simulink model "Control_Logic_e"  (R2021a)
settings: Solver=FixedStepAuto  StartTime=Start_time  StopTime=Stop_time  FixedStep=Sample_time  RelTol=1e-3
undefined symbols (not defined in the file or in its folder): Aset_N1, Aset_N10, Aset_N11, Aset_N12, Aset_N2, Aset_N3, Aset_N4, Aset_N5, Aset_N6, Aset_N7, Aset_N8, Aset_N9, Dset_N1, Dset_N2, Sample_time
(part 2 of 3)

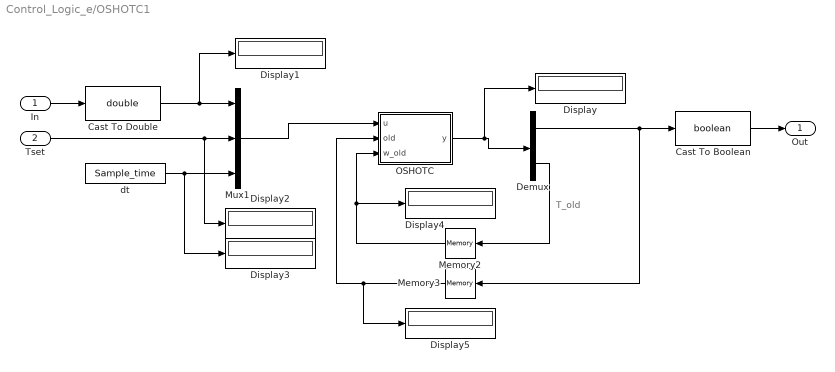
== system Control_Logic_e/OSHOTC1 ==
  note: T_old
  In : Inport
  Tset : Inport  Port=2
  Cast To Boolean : DataTypeConversion  OutDataTypeStr=boolean
  Cast To Double : DataTypeConversion  OutDataTypeStr=double
  Demux : Demux  Outputs=2
  Display{,1..5} (6 alike) : Display
  Memory2 : Memory  InheritSampleTime=on
  Memory3 : Memory  InheritSampleTime=on  LinearizeAsDelay=on
  Mux1 : Mux  Inputs=3
  OSHOTC : MATLAB Function  TreatAsAtomicUnit=on
  dt : Constant  Value=Sample_time  OutDataTypeStr=double  SampleTime=Sample_time
  Out : Outport  VectorParamsAs1DForOutWhenUnconnected=off
  wires:
  OSHOTC/1(y) -> Display/1, Demux/1
  Demux/1 -> Memory3/1, Cast To Boolean/1
  Cast To Boolean/1 -> Out/1
  Mux1/1 -> OSHOTC/1(u)
  Demux/2 -> Memory2/1
  Memory2/1 -> Display4/1, OSHOTC/3(w_old)
  dt/1 -> Display3/1, Mux1/3
  Tset/1 -> Display2/1, Mux1/2
  Memory3/1 -> Display5/1, OSHOTC/2(old)
  In/1 -> Cast To Double/1
  Cast To Double/1 -> Display1/1, Mux1/1

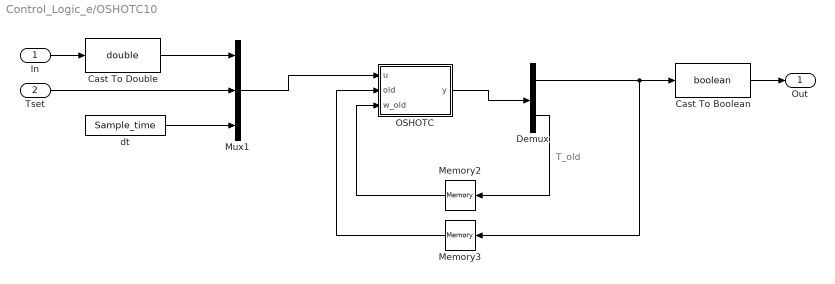
== system Control_Logic_e/OSHOTC10 ==
  note: T_old
  In : Inport
  Tset : Inport  Port=2
  Cast To Boolean : DataTypeConversion  OutDataTypeStr=boolean
  Cast To Double : DataTypeConversion  OutDataTypeStr=double
  Demux : Demux  Outputs=2
  Memory2 : Memory  InheritSampleTime=on
  Memory3 : Memory  InheritSampleTime=on  LinearizeAsDelay=on
  Mux1 : Mux  Inputs=3
  OSHOTC : MATLAB Function  TreatAsAtomicUnit=on
  dt : Constant  Value=Sample_time  OutDataTypeStr=double  SampleTime=Sample_time
  Out : Outport  VectorParamsAs1DForOutWhenUnconnected=off
  wires:
  Cast To Double/1 -> Mux1/1
  In/1 -> Cast To Double/1
  Memory3/1 -> OSHOTC/2(old)
  Tset/1 -> Mux1/2
  dt/1 -> Mux1/3
  Memory2/1 -> OSHOTC/3(w_old)
  Demux/2 -> Memory2/1
  Mux1/1 -> OSHOTC/1(u)
  Cast To Boolean/1 -> Out/1
  Demux/1 -> Cast To Boolean/1, Memory3/1
  OSHOTC/1(y) -> Demux/1

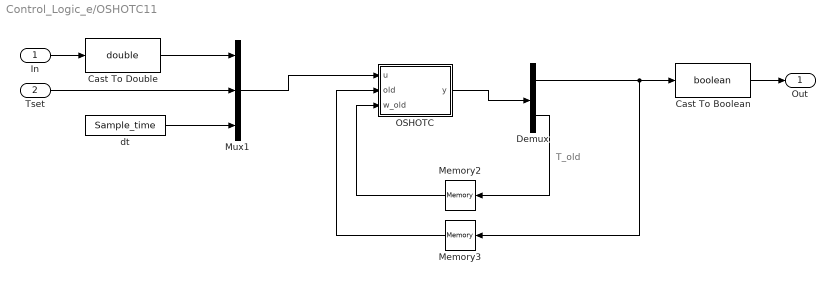
== system Control_Logic_e/OSHOTC11 ==
  note: T_old
  In : Inport
  Tset : Inport  Port=2
  Cast To Boolean : DataTypeConversion  OutDataTypeStr=boolean
  Cast To Double : DataTypeConversion  OutDataTypeStr=double
  Demux : Demux  Outputs=2
  Memory2 : Memory  InheritSampleTime=on
  Memory3 : Memory  InheritSampleTime=on  LinearizeAsDelay=on
  Mux1 : Mux  Inputs=3
  OSHOTC : MATLAB Function  TreatAsAtomicUnit=on
  dt : Constant  Value=Sample_time  OutDataTypeStr=double  SampleTime=Sample_time
  Out : Outport  VectorParamsAs1DForOutWhenUnconnected=off
  wires:
  OSHOTC/1(y) -> Demux/1
  Demux/1 -> Memory3/1, Cast To Boolean/1
  Cast To Boolean/1 -> Out/1
  Mux1/1 -> OSHOTC/1(u)
  Demux/2 -> Memory2/1
  Memory2/1 -> OSHOTC/3(w_old)
  dt/1 -> Mux1/3
  Tset/1 -> Mux1/2
  Memory3/1 -> OSHOTC/2(old)
  In/1 -> Cast To Double/1
  Cast To Double/1 -> Mux1/1

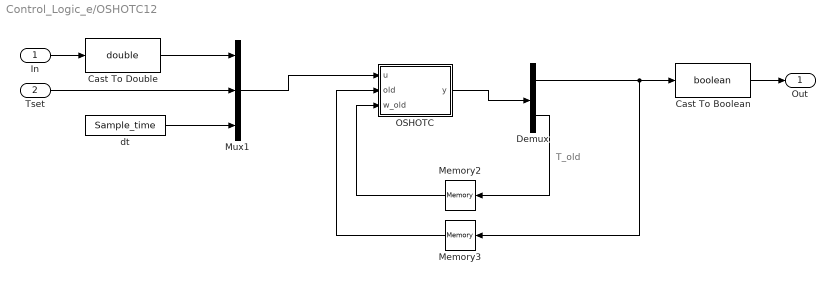
== system Control_Logic_e/OSHOTC12 ==
  note: T_old
  In : Inport
  Tset : Inport  Port=2
  Cast To Boolean : DataTypeConversion  OutDataTypeStr=boolean
  Cast To Double : DataTypeConversion  OutDataTypeStr=double
  Demux : Demux  Outputs=2
  Memory2 : Memory  InheritSampleTime=on
  Memory3 : Memory  InheritSampleTime=on  LinearizeAsDelay=on
  Mux1 : Mux  Inputs=3
  OSHOTC : MATLAB Function  TreatAsAtomicUnit=on
  dt : Constant  Value=Sample_time  OutDataTypeStr=double  SampleTime=Sample_time
  Out : Outport  VectorParamsAs1DForOutWhenUnconnected=off
  wires:
  OSHOTC/1(y) -> Demux/1
  Demux/1 -> Memory3/1, Cast To Boolean/1
  Cast To Boolean/1 -> Out/1
  Mux1/1 -> OSHOTC/1(u)
  Demux/2 -> Memory2/1
  Memory2/1 -> OSHOTC/3(w_old)
  dt/1 -> Mux1/3
  Tset/1 -> Mux1/2
  Memory3/1 -> OSHOTC/2(old)
  In/1 -> Cast To Double/1
  Cast To Double/1 -> Mux1/1

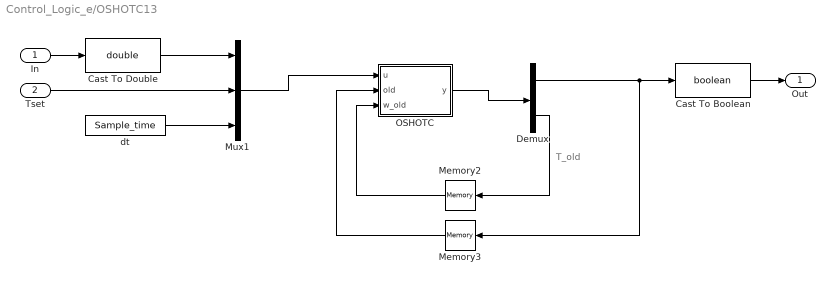
== system Control_Logic_e/OSHOTC13 ==
  note: T_old
  In : Inport
  Tset : Inport  Port=2
  Cast To Boolean : DataTypeConversion  OutDataTypeStr=boolean
  Cast To Double : DataTypeConversion  OutDataTypeStr=double
  Demux : Demux  Outputs=2
  Memory2 : Memory  InheritSampleTime=on
  Memory3 : Memory  InheritSampleTime=on  LinearizeAsDelay=on
  Mux1 : Mux  Inputs=3
  OSHOTC : MATLAB Function  TreatAsAtomicUnit=on
  dt : Constant  Value=Sample_time  OutDataTypeStr=double  SampleTime=Sample_time
  Out : Outport  VectorParamsAs1DForOutWhenUnconnected=off
  wires:
  OSHOTC/1(y) -> Demux/1
  Demux/1 -> Memory3/1, Cast To Boolean/1
  Cast To Boolean/1 -> Out/1
  Mux1/1 -> OSHOTC/1(u)
  Demux/2 -> Memory2/1
  Memory2/1 -> OSHOTC/3(w_old)
  dt/1 -> Mux1/3
  Tset/1 -> Mux1/2
  Memory3/1 -> OSHOTC/2(old)
  In/1 -> Cast To Double/1
  Cast To Double/1 -> Mux1/1

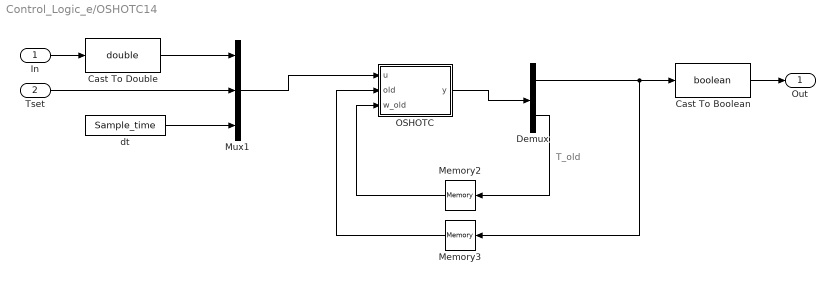
== system Control_Logic_e/OSHOTC14 ==
  note: T_old
  In : Inport
  Tset : Inport  Port=2
  Cast To Boolean : DataTypeConversion  OutDataTypeStr=boolean
  Cast To Double : DataTypeConversion  OutDataTypeStr=double
  Demux : Demux  Outputs=2
  Memory2 : Memory  InheritSampleTime=on
  Memory3 : Memory  InheritSampleTime=on  LinearizeAsDelay=on
  Mux1 : Mux  Inputs=3
  OSHOTC : MATLAB Function  TreatAsAtomicUnit=on
  dt : Constant  Value=Sample_time  OutDataTypeStr=double  SampleTime=Sample_time
  Out : Outport  VectorParamsAs1DForOutWhenUnconnected=off
  wires:
  OSHOTC/1(y) -> Demux/1
  Demux/1 -> Memory3/1, Cast To Boolean/1
  Cast To Boolean/1 -> Out/1
  Mux1/1 -> OSHOTC/1(u)
  Demux/2 -> Memory2/1
  Memory2/1 -> OSHOTC/3(w_old)
  dt/1 -> Mux1/3
  Tset/1 -> Mux1/2
  Memory3/1 -> OSHOTC/2(old)
  In/1 -> Cast To Double/1
  Cast To Double/1 -> Mux1/1

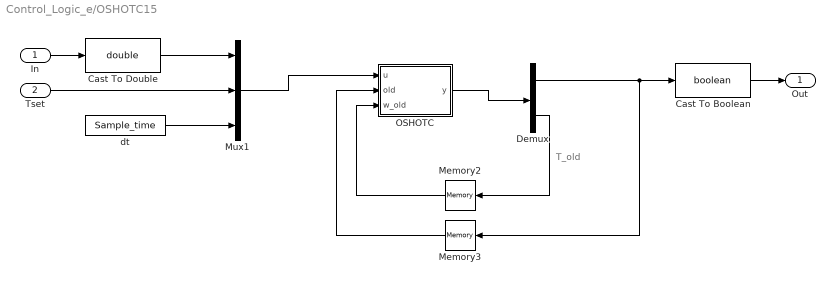
== system Control_Logic_e/OSHOTC15 ==
  note: T_old
  In : Inport
  Tset : Inport  Port=2
  Cast To Boolean : DataTypeConversion  OutDataTypeStr=boolean
  Cast To Double : DataTypeConversion  OutDataTypeStr=double
  Demux : Demux  Outputs=2
  Memory2 : Memory  InheritSampleTime=on
  Memory3 : Memory  InheritSampleTime=on  LinearizeAsDelay=on
  Mux1 : Mux  Inputs=3
  OSHOTC : MATLAB Function  TreatAsAtomicUnit=on
  dt : Constant  Value=Sample_time  OutDataTypeStr=double  SampleTime=Sample_time
  Out : Outport  VectorParamsAs1DForOutWhenUnconnected=off
  wires:
  OSHOTC/1(y) -> Demux/1
  Demux/1 -> Memory3/1, Cast To Boolean/1
  Cast To Boolean/1 -> Out/1
  Mux1/1 -> OSHOTC/1(u)
  Demux/2 -> Memory2/1
  Memory2/1 -> OSHOTC/3(w_old)
  dt/1 -> Mux1/3
  Tset/1 -> Mux1/2
  Memory3/1 -> OSHOTC/2(old)
  In/1 -> Cast To Double/1
  Cast To Double/1 -> Mux1/1

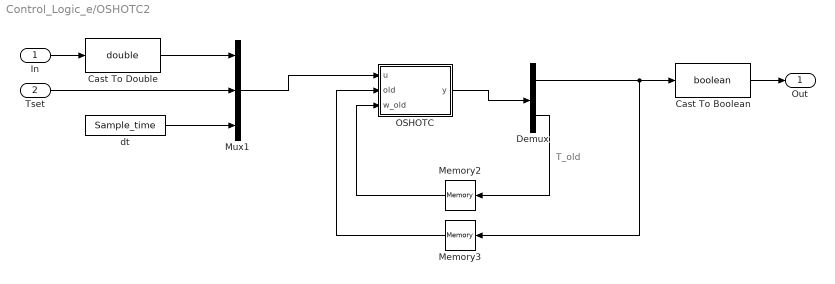
== system Control_Logic_e/OSHOTC2 ==
  note: T_old
  In : Inport
  Tset : Inport  Port=2
  Cast To Boolean : DataTypeConversion  OutDataTypeStr=boolean
  Cast To Double : DataTypeConversion  OutDataTypeStr=double
  Demux : Demux  Outputs=2
  Memory2 : Memory  InheritSampleTime=on
  Memory3 : Memory  InheritSampleTime=on  LinearizeAsDelay=on
  Mux1 : Mux  Inputs=3
  OSHOTC : MATLAB Function  TreatAsAtomicUnit=on
  dt : Constant  Value=Sample_time  OutDataTypeStr=double  SampleTime=Sample_time
  Out : Outport  VectorParamsAs1DForOutWhenUnconnected=off
  wires:
  OSHOTC/1(y) -> Demux/1
  Demux/1 -> Memory3/1, Cast To Boolean/1
  Cast To Boolean/1 -> Out/1
  Mux1/1 -> OSHOTC/1(u)
  Demux/2 -> Memory2/1
  Memory2/1 -> OSHOTC/3(w_old)
  dt/1 -> Mux1/3
  Tset/1 -> Mux1/2
  Memory3/1 -> OSHOTC/2(old)
  In/1 -> Cast To Double/1
  Cast To Double/1 -> Mux1/1

== system Control_Logic_e/OSHOTC3 ==
  note: T_old
  In : Inport
  Tset : Inport  Port=2
  Cast To Boolean : DataTypeConversion  OutDataTypeStr=boolean
  Cast To Double : DataTypeConversion  OutDataTypeStr=double
  Demux : Demux  Outputs=2
  Memory2 : Memory  InheritSampleTime=on
  Memory3 : Memory  InheritSampleTime=on  LinearizeAsDelay=on
  Mux1 : Mux  Inputs=3
  OSHOTC : MATLAB Function  TreatAsAtomicUnit=on
  dt : Constant  Value=Sample_time  OutDataTypeStr=double  SampleTime=Sample_time
  Out : Outport  VectorParamsAs1DForOutWhenUnconnected=off
  wires:
  OSHOTC/1(y) -> Demux/1
  Demux/1 -> Memory3/1, Cast To Boolean/1
  Cast To Boolean/1 -> Out/1
  Mux1/1 -> OSHOTC/1(u)
  Demux/2 -> Memory2/1
  Memory2/1 -> OSHOTC/3(w_old)
  dt/1 -> Mux1/3
  Tset/1 -> Mux1/2
  Memory3/1 -> OSHOTC/2(old)
  In/1 -> Cast To Double/1
  Cast To Double/1 -> Mux1/1

== system Control_Logic_e/OSHOTC4 ==
  note: T_old
  In : Inport
  Tset : Inport  Port=2
  Cast To Boolean : DataTypeConversion  OutDataTypeStr=boolean
  Cast To Double : DataTypeConversion  OutDataTypeStr=double
  Demux : Demux  Outputs=2
  Memory2 : Memory  InheritSampleTime=on
  Memory3 : Memory  InheritSampleTime=on  LinearizeAsDelay=on
  Mux1 : Mux  Inputs=3
  OSHOTC : MATLAB Function  TreatAsAtomicUnit=on
  dt : Constant  Value=Sample_time  OutDataTypeStr=double  SampleTime=Sample_time
  Out : Outport  VectorParamsAs1DForOutWhenUnconnected=off
  wires:
  OSHOTC/1(y) -> Demux/1
  Demux/1 -> Memory3/1, Cast To Boolean/1
  Cast To Boolean/1 -> Out/1
  Mux1/1 -> OSHOTC/1(u)
  Demux/2 -> Memory2/1
  Memory2/1 -> OSHOTC/3(w_old)
  dt/1 -> Mux1/3
  Tset/1 -> Mux1/2
  Memory3/1 -> OSHOTC/2(old)
  In/1 -> Cast To Double/1
  Cast To Double/1 -> Mux1/1

== system Control_Logic_e/OSHOTC5 ==
  note: T_old
  In : Inport
  Tset : Inport  Port=2
  Cast To Boolean : DataTypeConversion  OutDataTypeStr=boolean
  Cast To Double : DataTypeConversion  OutDataTypeStr=double
  Demux : Demux  Outputs=2
  Memory2 : Memory  InheritSampleTime=on
  Memory3 : Memory  InheritSampleTime=on  LinearizeAsDelay=on
  Mux1 : Mux  Inputs=3
  OSHOTC : MATLAB Function  TreatAsAtomicUnit=on
  dt : Constant  Value=Sample_time  OutDataTypeStr=double  SampleTime=Sample_time
  Out : Outport  VectorParamsAs1DForOutWhenUnconnected=off
  wires:
  OSHOTC/1(y) -> Demux/1
  Demux/1 -> Memory3/1, Cast To Boolean/1
  Cast To Boolean/1 -> Out/1
  Mux1/1 -> OSHOTC/1(u)
  Demux/2 -> Memory2/1
  Memory2/1 -> OSHOTC/3(w_old)
  dt/1 -> Mux1/3
  Tset/1 -> Mux1/2
  Memory3/1 -> OSHOTC/2(old)
  In/1 -> Cast To Double/1
  Cast To Double/1 -> Mux1/1

== system Control_Logic_e/OSHOTC6 ==
  note: T_old
  In : Inport
  Tset : Inport  Port=2
  Cast To Boolean : DataTypeConversion  OutDataTypeStr=boolean
  Cast To Double : DataTypeConversion  OutDataTypeStr=double
  Demux : Demux  Outputs=2
  Memory2 : Memory  InheritSampleTime=on
  Memory3 : Memory  InheritSampleTime=on  LinearizeAsDelay=on
  Mux1 : Mux  Inputs=3
  OSHOTC : MATLAB Function  TreatAsAtomicUnit=on
  dt : Constant  Value=Sample_time  OutDataTypeStr=double  SampleTime=Sample_time
  Out : Outport  VectorParamsAs1DForOutWhenUnconnected=off
  wires:
  OSHOTC/1(y) -> Demux/1
  Demux/1 -> Memory3/1, Cast To Boolean/1
  Cast To Boolean/1 -> Out/1
  Mux1/1 -> OSHOTC/1(u)
  Demux/2 -> Memory2/1
  Memory2/1 -> OSHOTC/3(w_old)
  dt/1 -> Mux1/3
  Tset/1 -> Mux1/2
  Memory3/1 -> OSHOTC/2(old)
  In/1 -> Cast To Double/1
  Cast To Double/1 -> Mux1/1

== system Control_Logic_e/OSHOTC7 ==
  note: T_old
  In : Inport
  Tset : Inport  Port=2
  Cast To Boolean : DataTypeConversion  OutDataTypeStr=boolean
  Cast To Double : DataTypeConversion  OutDataTypeStr=double
  Demux : Demux  Outputs=2
  Memory2 : Memory  InheritSampleTime=on
  Memory3 : Memory  InheritSampleTime=on  LinearizeAsDelay=on
  Mux1 : Mux  Inputs=3
  OSHOTC : MATLAB Function  TreatAsAtomicUnit=on
  dt : Constant  Value=Sample_time  OutDataTypeStr=double  SampleTime=Sample_time
  Out : Outport  VectorParamsAs1DForOutWhenUnconnected=off
  wires:
  OSHOTC/1(y) -> Demux/1
  Demux/1 -> Memory3/1, Cast To Boolean/1
  Cast To Boolean/1 -> Out/1
  Mux1/1 -> OSHOTC/1(u)
  Demux/2 -> Memory2/1
  Memory2/1 -> OSHOTC/3(w_old)
  dt/1 -> Mux1/3
  Tset/1 -> Mux1/2
  Memory3/1 -> OSHOTC/2(old)
  In/1 -> Cast To Double/1
  Cast To Double/1 -> Mux1/1

== system Control_Logic_e/OSHOTC8 ==
  note: T_old
  In : Inport
  Tset : Inport  Port=2
  Cast To Boolean : DataTypeConversion  OutDataTypeStr=boolean
  Cast To Double : DataTypeConversion  OutDataTypeStr=double
  Demux : Demux  Outputs=2
  Memory2 : Memory  InheritSampleTime=on
  Memory3 : Memory  InheritSampleTime=on  LinearizeAsDelay=on
  Mux1 : Mux  Inputs=3
  OSHOTC : MATLAB Function  TreatAsAtomicUnit=on
  dt : Constant  Value=Sample_time  OutDataTypeStr=double  SampleTime=Sample_time
  Out : Outport  VectorParamsAs1DForOutWhenUnconnected=off
  wires:
  OSHOTC/1(y) -> Demux/1
  Demux/1 -> Memory3/1, Cast To Boolean/1
  Cast To Boolean/1 -> Out/1
  Mux1/1 -> OSHOTC/1(u)
  Demux/2 -> Memory2/1
  Memory2/1 -> OSHOTC/3(w_old)
  dt/1 -> Mux1/3
  Tset/1 -> Mux1/2
  Memory3/1 -> OSHOTC/2(old)
  In/1 -> Cast To Double/1
  Cast To Double/1 -> Mux1/1

== system Control_Logic_e/OSHOTC9 ==
  note: T_old
  In : Inport
  Tset : Inport  Port=2
  Cast To Boolean : DataTypeConversion  OutDataTypeStr=boolean
  Cast To Double : DataTypeConversion  OutDataTypeStr=double
  Demux : Demux  Outputs=2
  Memory2 : Memory  InheritSampleTime=on
  Memory3 : Memory  InheritSampleTime=on  LinearizeAsDelay=on
  Mux1 : Mux  Inputs=3
  OSHOTC : MATLAB Function  TreatAsAtomicUnit=on
  dt : Constant  Value=Sample_time  OutDataTypeStr=double  SampleTime=Sample_time
  Out : Outport  VectorParamsAs1DForOutWhenUnconnected=off
  wires:
  OSHOTC/1(y) -> Demux/1
  Demux/1 -> Memory3/1, Cast To Boolean/1
  Cast To Boolean/1 -> Out/1
  Mux1/1 -> OSHOTC/1(u)
  Demux/2 -> Memory2/1
  Memory2/1 -> OSHOTC/3(w_old)
  dt/1 -> Mux1/3
  Tset/1 -> Mux1/2
  Memory3/1 -> OSHOTC/2(old)
  In/1 -> Cast To Double/1
  Cast To Double/1 -> Mux1/1

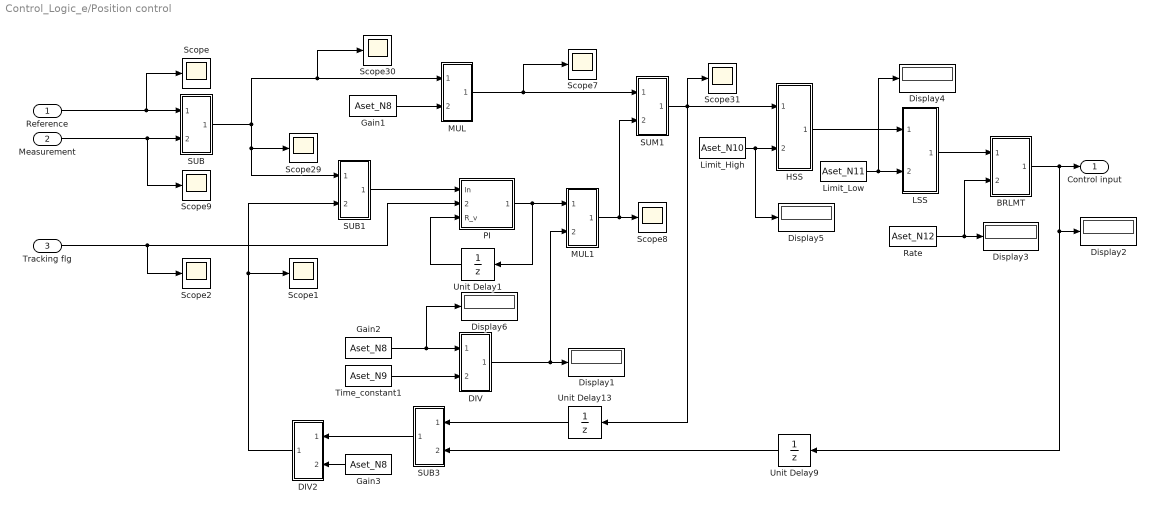
== system Control_Logic_e/Position control ==
  Reference : Inport
  Measurement : Inport  Port=2
  Tracking flg : Inport  Port=3
  BRLMT : Subsystem
  DIV : Subsystem
  DIV2 : Subsystem
  Display{1..6} (6 alike) : Display
  Gain1 : Constant  Value=Aset_N8  OutDataTypeStr=double  SampleTime=Sample_time
  Gain2 : Constant  Value=Aset_N8  OutDataTypeStr=double  SampleTime=Sample_time
  Gain3 : Constant  Value=Aset_N8  OutDataTypeStr=double  SampleTime=Sample_time
  HSS : Subsystem
  LSS : Subsystem
  Limit_High : Constant  Value=Aset_N10  OutDataTypeStr=double  SampleTime=Sample_time
  Limit_Low : Constant  Value=Aset_N11  OutDataTypeStr=double  SampleTime=Sample_time
  MUL : Subsystem
  MUL1 : Subsystem
  PI : Subsystem
  Rate : Constant  Value=Aset_N12  OutDataTypeStr=double  SampleTime=Sample_time
  SUB : Subsystem
  SUB1 : Subsystem
  SUB3 : Subsystem
  SUM1 : Subsystem
  Scope{,1..2,7..9,29..31} (9 alike) : Scope
  Time_constant1 : Constant  Value=Aset_N9  OutDataTypeStr=double  SampleTime=Sample_time
  Unit Delay1 : UnitDelay  SampleTime=Sample_time  HasFrameUpgradeWarning=on
  Unit Delay13 : UnitDelay  SampleTime=Sample_time  HasFrameUpgradeWarning=on
  Unit Delay9 : UnitDelay  SampleTime=Sample_time  HasFrameUpgradeWarning=on
  Control input : Outport  VectorParamsAs1DForOutWhenUnconnected=off
  wires:
  SUM1/1(Out) -> HSS/1(In1), Unit Delay13/1, Scope31/1
  Measurement/1 -> SUB/2(In2), Scope9/1
  SUB/1(Out) -> Scope30/1, MUL/1(In1), SUB1/1(In1), Scope29/1
  Unit Delay13/1 -> SUB3/1(In1)
  MUL/1(Out) -> Scope7/1, SUM1/1(In1)
  SUB3/1(Out) -> DIV2/1(In1)
  SUB1/1(Out) -> PI/1(In)
  Gain1/1 -> MUL/2(In2)
  LSS/1(Out1) -> BRLMT/1(In1)
  Reference/1 -> SUB/1(In1), Scope/1
  Gain3/1 -> DIV2/2(In2)
  Limit_Low/1 -> LSS/2(In2), Display4/1
  Tracking flg/1 -> PI/2(Reset), Scope2/1
  PI/1(Out1) -> MUL1/1(In1), Unit Delay1/1
  Limit_High/1 -> HSS/2(In2), Display5/1
  MUL1/1(Out) -> SUM1/2(In2), Scope8/1
  BRLMT/1(Out1) -> Unit Delay9/1, Display2/1, Control input/1
  Time_constant1/1 -> DIV/2(In2)
  Gain2/1 -> DIV/1(In1), Display6/1
  HSS/1(Out1) -> LSS/1(In1)
  DIV2/1(Out1) -> SUB1/2(In2), Scope1/1
  Unit Delay9/1 -> SUB3/2(In2)
  DIV/1(Out1) -> MUL1/2(In2), Display1/1
  Rate/1 -> BRLMT/2(In2), Display3/1
  Unit Delay1/1 -> PI/3(R_v)

== system Control_Logic_e/SUB ==
  In1 : Inport
  In2 : Inport  Port=2
  Mux : Mux  Inputs=2
  SUB : MATLAB Function  TreatAsAtomicUnit=on
  Out : Outport  VectorParamsAs1DForOutWhenUnconnected=off
  wires:
  In2/1 -> Mux/2
  SUB/1(y) -> Out/1
  Mux/1 -> SUB/1(u)
  In1/1 -> Mux/1

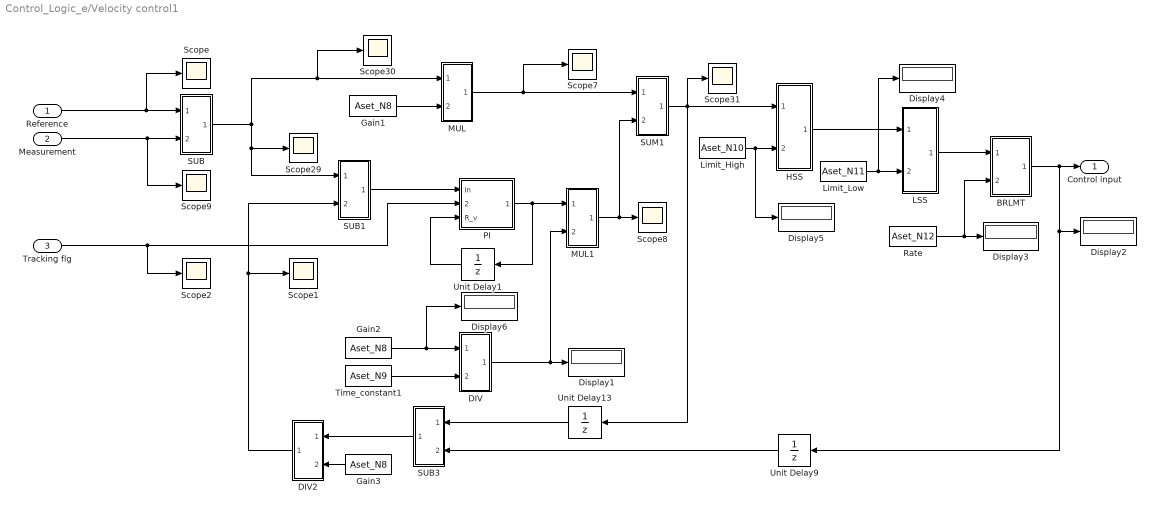
== system Control_Logic_e/Velocity control1 ==
  Reference : Inport
  Measurement : Inport  Port=2
  Tracking flg : Inport  Port=3
  BRLMT : Subsystem
  DIV : Subsystem
  DIV2 : Subsystem
  Display{1..6} (6 alike) : Display
  Gain1 : Constant  Value=Aset_N8  OutDataTypeStr=double  SampleTime=Sample_time
  Gain2 : Constant  Value=Aset_N8  OutDataTypeStr=double  SampleTime=Sample_time
  Gain3 : Constant  Value=Aset_N8  OutDataTypeStr=double  SampleTime=Sample_time
  HSS : Subsystem
  LSS : Subsystem
  Limit_High : Constant  Value=Aset_N10  OutDataTypeStr=double  SampleTime=Sample_time
  Limit_Low : Constant  Value=Aset_N11  OutDataTypeStr=double  SampleTime=Sample_time
  MUL : Subsystem
  MUL1 : Subsystem
  PI : Subsystem
  Rate : Constant  Value=Aset_N12  OutDataTypeStr=double  SampleTime=Sample_time
  SUB : Subsystem
  SUB1 : Subsystem
  SUB3 : Subsystem
  SUM1 : Subsystem
  Scope{,1..2,7..9,29..31} (9 alike) : Scope
  Time_constant1 : Constant  Value=Aset_N9  OutDataTypeStr=double  SampleTime=Sample_time
  Unit Delay1 : UnitDelay  SampleTime=Sample_time  HasFrameUpgradeWarning=on
  Unit Delay13 : UnitDelay  SampleTime=Sample_time  HasFrameUpgradeWarning=on
  Unit Delay9 : UnitDelay  SampleTime=Sample_time  HasFrameUpgradeWarning=on
  Control input : Outport  VectorParamsAs1DForOutWhenUnconnected=off
  wires:
  Unit Delay1/1 -> PI/3(R_v)
  Rate/1 -> Display3/1, BRLMT/2(In2)
  DIV/1(Out1) -> Display1/1, MUL1/2(In2)
  Unit Delay9/1 -> SUB3/2(In2)
  DIV2/1(Out1) -> Scope1/1, SUB1/2(In2)
  HSS/1(Out1) -> LSS/1(In1)
  Gain2/1 -> Display6/1, DIV/1(In1)
  Time_constant1/1 -> DIV/2(In2)
  BRLMT/1(Out1) -> Control input/1, Display2/1, Unit Delay9/1
  MUL1/1(Out) -> Scope8/1, SUM1/2(In2)
  Limit_High/1 -> Display5/1, HSS/2(In2)
  PI/1(Out1) -> Unit Delay1/1, MUL1/1(In1)
  Tracking flg/1 -> Scope2/1, PI/2(Reset)
  Limit_Low/1 -> Display4/1, LSS/2(In2)
  Gain3/1 -> DIV2/2(In2)
  Reference/1 -> Scope/1, SUB/1(In1)
  LSS/1(Out1) -> BRLMT/1(In1)
  Gain1/1 -> MUL/2(In2)
  SUB1/1(Out) -> PI/1(In)
  SUB3/1(Out) -> DIV2/1(In1)
  MUL/1(Out) -> SUM1/1(In1), Scope7/1
  Unit Delay13/1 -> SUB3/1(In1)
  SUB/1(Out) -> Scope29/1, SUB1/1(In1), MUL/1(In1), Scope30/1
  Measurement/1 -> Scope9/1, SUB/2(In2)
  SUM1/1(Out) -> Scope31/1, Unit Delay13/1, HSS/1(In1)

== system Control_Logic_e/Position control/BRLMT ==
  In1 : Inport
  In2 : Inport  Port=2
  BRLMT : MATLAB Function  TreatAsAtomicUnit=on
  Display : Display
  Memory : Memory  InheritSampleTime=on  LinearizeMemory=on  LinearizeAsDelay=on
  Mux1 : Mux  Inputs=3
  dt : Constant  Value=Sample_time  OutDataTypeStr=double  SampleTime=Sample_time
  Out1 : Outport  VectorParamsAs1DForOutWhenUnconnected=off
  wires:
  In1/1 -> Mux1/1
  Mux1/1 -> Display/1, BRLMT/1(u)
  BRLMT/1(y) -> Out1/1, Memory/1
  Memory/1 -> BRLMT/2(old)
  In2/1 -> Mux1/2
  dt/1 -> Mux1/3

== system Control_Logic_e/Position control/DIV ==
  In1 : Inport
  In2 : Inport  Port=2
  DIV : MATLAB Function  TreatAsAtomicUnit=on
  Display : Display
  Display1 : Display
  FlowMax1 : Constant  Value=3.402823e+38  OutDataTypeStr=double  SampleTime=Sample_time
  Mux : Mux  Inputs=3
  Out1 : Outport  VectorParamsAs1DForOutWhenUnconnected=off
  wires:
  FlowMax1/1 -> Mux/3
  In1/1 -> Mux/1, Display/1
  Mux/1 -> DIV/1(u)
  DIV/1(y) -> Out1/1
  In2/1 -> Display1/1, Mux/2

== system Control_Logic_e/Position control/DIV2 ==
  In1 : Inport
  In2 : Inport  Port=2
  DIV : MATLAB Function  TreatAsAtomicUnit=on
  Display : Display
  Display1 : Display
  FlowMax1 : Constant  Value=3.402823e+38  OutDataTypeStr=double  SampleTime=Sample_time
  Mux : Mux  Inputs=3
  Out1 : Outport  VectorParamsAs1DForOutWhenUnconnected=off
  wires:
  FlowMax1/1 -> Mux/3
  In1/1 -> Mux/1, Display/1
  Mux/1 -> DIV/1(u)
  DIV/1(y) -> Out1/1
  In2/1 -> Display1/1, Mux/2

== system Control_Logic_e/Position control/HSS ==
  In1 : Inport
  In2 : Inport  Port=2
  HSS : MATLAB Function  TreatAsAtomicUnit=on
  Mux : Mux  Inputs=2
  Out1 : Outport  VectorParamsAs1DForOutWhenUnconnected=off
  wires:
  HSS/1(y) -> Out1/1
  In1/1 -> Mux/1
  In2/1 -> Mux/2
  Mux/1 -> HSS/1(u)

== system Control_Logic_e/Position control/LSS ==
  In1 : Inport
  In2 : Inport  Port=2
  LSS : MATLAB Function  TreatAsAtomicUnit=on
  Mux : Mux  Inputs=2
  Out1 : Outport  VectorParamsAs1DForOutWhenUnconnected=off
  wires:
  LSS/1(y) -> Out1/1
  Mux/1 -> LSS/1(u)
  In1/1 -> Mux/1
  In2/1 -> Mux/2

== system Control_Logic_e/Position control/MUL ==
  In1 : Inport
  In2 : Inport  Port=2
  MUL : MATLAB Function  TreatAsAtomicUnit=on
  Mux : Mux  Inputs=2
  Out : Outport  VectorParamsAs1DForOutWhenUnconnected=off
  wires:
  In1/1 -> Mux/1
  Mux/1 -> MUL/1(u)
  MUL/1(y) -> Out/1
  In2/1 -> Mux/2

== system Control_Logic_e/Position control/MUL1 ==
  In1 : Inport
  In2 : Inport  Port=2
  MUL : MATLAB Function  TreatAsAtomicUnit=on
  Mux : Mux  Inputs=2
  Out : Outport  VectorParamsAs1DForOutWhenUnconnected=off
  wires:
  In1/1 -> Mux/1
  Mux/1 -> MUL/1(u)
  MUL/1(y) -> Out/1
  In2/1 -> Mux/2

== system Control_Logic_e/Position control/PI ==
  In : Inport
  Reset : Inport  Port=2
  R_v : Inport  Port=3
  Cast To Double : DataTypeConversion  OutDataTypeStr=double
  Memory : Memory  InheritSampleTime=on
  Mux : Mux
  PI : MATLAB Function  TreatAsAtomicUnit=on
  dt : Constant  Value=Sample_time  OutDataTypeStr=double  SampleTime=Sample_time
  Out1 : Outport  VectorParamsAs1DForOutWhenUnconnected=off
  wires:
  In/1 -> Mux/1
  Reset/1 -> Cast To Double/1
  PI/1(y) -> Out1/1, Memory/1
  Mux/1 -> PI/1(u)
  R_v/1 -> Mux/3
  dt/1 -> Mux/4
  Cast To Double/1 -> Mux/2
  Memory/1 -> PI/2(old)

== system Control_Logic_e/Position control/SUB ==
  In1 : Inport
  In2 : Inport  Port=2
  Mux : Mux  Inputs=2
  SUB : MATLAB Function  TreatAsAtomicUnit=on
  Out : Outport  VectorParamsAs1DForOutWhenUnconnected=off
  wires:
  In2/1 -> Mux/2
  SUB/1(y) -> Out/1
  Mux/1 -> SUB/1(u)
  In1/1 -> Mux/1

== system Control_Logic_e/Position control/SUB1 ==
  In1 : Inport
  In2 : Inport  Port=2
  Mux : Mux  Inputs=2
  SUB : MATLAB Function  TreatAsAtomicUnit=on
  Out : Outport  VectorParamsAs1DForOutWhenUnconnected=off
  wires:
  In1/1 -> Mux/1
  Mux/1 -> SUB/1(u)
  SUB/1(y) -> Out/1
  In2/1 -> Mux/2

== system Control_Logic_e/Position control/SUB3 ==
  In1 : Inport
  In2 : Inport  Port=2
  Mux : Mux  Inputs=2
  SUB : MATLAB Function  TreatAsAtomicUnit=on
  Out : Outport  VectorParamsAs1DForOutWhenUnconnected=off
  wires:
  In2/1 -> Mux/2
  SUB/1(y) -> Out/1
  Mux/1 -> SUB/1(u)
  In1/1 -> Mux/1

== system Control_Logic_e/Position control/SUM1 ==
  In1 : Inport
  In2 : Inport  Port=2
  Mux : Mux  Inputs=2
  SUM : MATLAB Function  TreatAsAtomicUnit=on
  Out : Outport  VectorParamsAs1DForOutWhenUnconnected=off
  wires:
  Mux/1 -> SUM/1(u)
  SUM/1(y) -> Out/1
  In1/1 -> Mux/1
  In2/1 -> Mux/2

== system Control_Logic_e/Velocity control1/BRLMT ==
  In1 : Inport
  In2 : Inport  Port=2
  BRLMT : MATLAB Function  TreatAsAtomicUnit=on
  Display : Display
  Memory : Memory  InheritSampleTime=on  LinearizeMemory=on  LinearizeAsDelay=on
  Mux1 : Mux  Inputs=3
  dt : Constant  Value=Sample_time  OutDataTypeStr=double  SampleTime=Sample_time
  Out1 : Outport  VectorParamsAs1DForOutWhenUnconnected=off
  wires:
  dt/1 -> Mux1/3
  In2/1 -> Mux1/2
  Memory/1 -> BRLMT/2(old)
  BRLMT/1(y) -> Memory/1, Out1/1
  Mux1/1 -> BRLMT/1(u), Display/1
  In1/1 -> Mux1/1

== system Control_Logic_e/Velocity control1/DIV ==
  In1 : Inport
  In2 : Inport  Port=2
  DIV : MATLAB Function  TreatAsAtomicUnit=on
  Display : Display
  Display1 : Display
  FlowMax1 : Constant  Value=3.402823e+38  OutDataTypeStr=double  SampleTime=Sample_time
  Mux : Mux  Inputs=3
  Out1 : Outport  VectorParamsAs1DForOutWhenUnconnected=off
  wires:
  In2/1 -> Mux/2, Display1/1
  DIV/1(y) -> Out1/1
  Mux/1 -> DIV/1(u)
  In1/1 -> Display/1, Mux/1
  FlowMax1/1 -> Mux/3

== system Control_Logic_e/Velocity control1/DIV2 ==
  In1 : Inport
  In2 : Inport  Port=2
  DIV : MATLAB Function  TreatAsAtomicUnit=on
  Display : Display
  Display1 : Display
  FlowMax1 : Constant  Value=3.402823e+38  OutDataTypeStr=double  SampleTime=Sample_time
  Mux : Mux  Inputs=3
  Out1 : Outport  VectorParamsAs1DForOutWhenUnconnected=off
  wires:
  In2/1 -> Mux/2, Display1/1
  DIV/1(y) -> Out1/1
  Mux/1 -> DIV/1(u)
  In1/1 -> Display/1, Mux/1
  FlowMax1/1 -> Mux/3

== system Control_Logic_e/Velocity control1/HSS ==
  In1 : Inport
  In2 : Inport  Port=2
  HSS : MATLAB Function  TreatAsAtomicUnit=on
  Mux : Mux  Inputs=2
  Out1 : Outport  VectorParamsAs1DForOutWhenUnconnected=off
  wires:
  Mux/1 -> HSS/1(u)
  In2/1 -> Mux/2
  In1/1 -> Mux/1
  HSS/1(y) -> Out1/1

== system Control_Logic_e/Velocity control1/LSS ==
  In1 : Inport
  In2 : Inport  Port=2
  LSS : MATLAB Function  TreatAsAtomicUnit=on
  Mux : Mux  Inputs=2
  Out1 : Outport  VectorParamsAs1DForOutWhenUnconnected=off
  wires:
  In2/1 -> Mux/2
  In1/1 -> Mux/1
  Mux/1 -> LSS/1(u)
  LSS/1(y) -> Out1/1

== system Control_Logic_e/Velocity control1/MUL ==
  In1 : Inport
  In2 : Inport  Port=2
  MUL : MATLAB Function  TreatAsAtomicUnit=on
  Mux : Mux  Inputs=2
  Out : Outport  VectorParamsAs1DForOutWhenUnconnected=off
  wires:
  In2/1 -> Mux/2
  MUL/1(y) -> Out/1
  Mux/1 -> MUL/1(u)
  In1/1 -> Mux/1

== system Control_Logic_e/Velocity control1/MUL1 ==
  In1 : Inport
  In2 : Inport  Port=2
  MUL : MATLAB Function  TreatAsAtomicUnit=on
  Mux : Mux  Inputs=2
  Out : Outport  VectorParamsAs1DForOutWhenUnconnected=off
  wires:
  In2/1 -> Mux/2
  MUL/1(y) -> Out/1
  Mux/1 -> MUL/1(u)
  In1/1 -> Mux/1

== system Control_Logic_e/Velocity control1/PI ==
  In : Inport
  Reset : Inport  Port=2
  R_v : Inport  Port=3
  Cast To Double : DataTypeConversion  OutDataTypeStr=double
  Memory : Memory  InheritSampleTime=on
  Mux : Mux
  PI : MATLAB Function  TreatAsAtomicUnit=on
  dt : Constant  Value=Sample_time  OutDataTypeStr=double  SampleTime=Sample_time
  Out1 : Outport  VectorParamsAs1DForOutWhenUnconnected=off
  wires:
  Memory/1 -> PI/2(old)
  Cast To Double/1 -> Mux/2
  dt/1 -> Mux/4
  R_v/1 -> Mux/3
  Mux/1 -> PI/1(u)
  PI/1(y) -> Memory/1, Out1/1
  Reset/1 -> Cast To Double/1
  In/1 -> Mux/1

== system Control_Logic_e/Velocity control1/SUB ==
  In1 : Inport
  In2 : Inport  Port=2
  Mux : Mux  Inputs=2
  SUB : MATLAB Function  TreatAsAtomicUnit=on
  Out : Outport  VectorParamsAs1DForOutWhenUnconnected=off
  wires:
  In1/1 -> Mux/1
  Mux/1 -> SUB/1(u)
  SUB/1(y) -> Out/1
  In2/1 -> Mux/2

== system Control_Logic_e/Velocity control1/SUB1 ==
  In1 : Inport
  In2 : Inport  Port=2
  Mux : Mux  Inputs=2
  SUB : MATLAB Function  TreatAsAtomicUnit=on
  Out : Outport  VectorParamsAs1DForOutWhenUnconnected=off
  wires:
  In2/1 -> Mux/2
  SUB/1(y) -> Out/1
  Mux/1 -> SUB/1(u)
  In1/1 -> Mux/1

== system Control_Logic_e/Velocity control1/SUB3 ==
  In1 : Inport
  In2 : Inport  Port=2
  Mux : Mux  Inputs=2
  SUB : MATLAB Function  TreatAsAtomicUnit=on
  Out : Outport  VectorParamsAs1DForOutWhenUnconnected=off
  wires:
  In1/1 -> Mux/1
  Mux/1 -> SUB/1(u)
  SUB/1(y) -> Out/1
  In2/1 -> Mux/2

== system Control_Logic_e/Velocity control1/SUM1 ==
  In1 : Inport
  In2 : Inport  Port=2
  Mux : Mux  Inputs=2
  SUM : MATLAB Function  TreatAsAtomicUnit=on
  Out : Outport  VectorParamsAs1DForOutWhenUnconnected=off
  wires:
  In2/1 -> Mux/2
  In1/1 -> Mux/1
  SUM/1(y) -> Out/1
  Mux/1 -> SUM/1(u)

== matlab function Control_Logic_e/NOT1/NOT ==
  data: u input; y output
%反転
function y  = NOT(u)
    y = 0;
    ud = logical(u(1));
    if ud == false        
        temp = true;
    else
        temp = false;
    end
    y = double(temp);
end

== matlab function Control_Logic_e/NOT7/NOT ==
  data: u input; y output
%反転
function y  = NOT(u)
    y = 0;
    ud = logical(u(1));
    if ud == false        
        temp = true;
    else
        temp = false;
    end
    y = double(temp);
end

== matlab function Control_Logic_e/AND13/AND ==
  data: u input; y output
% 論理積
function y  = AND(u)
   y = 0;
   dy = true;
   for i = 1:size(u,1)
    dy = logical(u(i)) & dy;
   end
    y = double(dy);
end

== matlab function Control_Logic_e/ANSW/MATLAB Function ==
  data: u input; y output
% 2位置(アナログ)スイッチ
%   u3入力がONならば、 y=x1(A入力を選択)
%   u3入力がOFFならば、 y=x2(B入力を選択)
%       u(2):A入力変数
%       u(3):B入力変数
%       u3=u(1):C入力変数
%       y : 出力変数
function y  = ANSW(u)
    y = 0;
    temp = logical(u(1));
    temp2 = 0;
    if temp ~= false
        temp2 = u(2);
    else
        temp2 = u(3); 
    end
    y = temp2;
end

== matlab function Control_Logic_e/ONDLC3/ONDLC ==
  data: u input; y output; old input; set input
% オンディレイ タイマ
%  xがONとなってからパラメータで設定した[sec]後にyがONとなる。
%  なお、xのON状態がパラメータで設定した[sec]続かずにOFF状態
%  へ戻った場合はyはOFF状態を継続する。
%       ud=u(1) :入力信号
%       set=u(2)：時定数
%       timc(1)=u(3)：計算刻み
%       timc(2)=u(4)：経過時間(前回値)
%       y : 出力信号
function y  = ONDLC(u, old, set)
    assignin('base','run_info',sprintf('%sOND#%f$',evalin('base','run_info'),u(2)));
       y=zeros(2,1);
       ud = logical(u(1));
       set=u(2);
       timc1=u(3);
       timc2=old(1);
    if ud == false
        temp = false;
        w = 0;
    else
        if timc2 < set 
            temp = false;
            w = timc2 + timc1;
        else
            temp = true;
            w = timc2;
        end
    end
    
    y(1)=double(temp);
    y(2)=w;
end

== matlab function Control_Logic_e/AND/AND ==
  data: u input; y output
% 論理積
function y  = AND(u)
   y = 0;
   dy = true;
   for i = 1:size(u,1)
    dy = logical(u(i)) & dy;
   end
    y = double(dy);
end

== matlab function Control_Logic_e/AND14/AND ==
  data: u input; y output
% 論理積
function y  = AND(u)
   y = 0;
   dy = true;
   for i = 1:size(u,1)
    dy = logical(u(i)) & dy;
   end
    y = double(dy);
end

== matlab function Control_Logic_e/OR2/MATLAB Function ==
  data: u input; y output
% 論理積
function y  = OR(u)
   y= 0;
   dy = false;
   for i = 1:size(u,1)
   dy = logical(u(i)) | dy;
   end
    y = double(dy);
end

== matlab function Control_Logic_e/AND2/AND ==
  data: u input; y output
% 論理積
function y  = AND(u)
   y = 0;
   dy = true;
   for i = 1:size(u,1)
    dy = logical(u(i)) & dy;
   end
    y = double(dy);
end

== matlab function Control_Logic_e/AND3/AND ==
  data: u input; y output
% 論理積
function y  = AND(u)
   y = 0;
   dy = true;
   for i = 1:size(u,1)
    dy = logical(u(i)) & dy;
   end
    y = double(dy);
end

== matlab function Control_Logic_e/NOT2/NOT ==
  data: u input; y output
%反転
function y  = NOT(u)
    y = 0;
    ud = logical(u(1));
    if ud == false        
        temp = true;
    else
        temp = false;
    end
    y = double(temp);
end

== matlab function Control_Logic_e/AND4/AND ==
  data: u input; y output
% 論理積
function y  = AND(u)
   y = 0;
   dy = true;
   for i = 1:size(u,1)
    dy = logical(u(i)) & dy;
   end
    y = double(dy);
end

== matlab function Control_Logic_e/AND6/AND ==
  data: u input; y output
% 論理積
function y  = AND(u)
   y = 0;
   dy = true;
   for i = 1:size(u,1)
    dy = logical(u(i)) & dy;
   end
    y = double(dy);
end

== matlab function Control_Logic_e/AND9/AND ==
  data: u input; y output
% 論理積
function y  = AND(u)
   y = 0;
   dy = true;
   for i = 1:size(u,1)
    dy = logical(u(i)) & dy;
   end
    y = double(dy);
end

== matlab function Control_Logic_e/AND10/AND ==
  data: u input; y output
% 論理積
function y  = AND(u)
   y = 0;
   dy = true;
   for i = 1:size(u,1)
    dy = logical(u(i)) & dy;
   end
    y = double(dy);
end

== matlab function Control_Logic_e/AND11/AND ==
  data: u input; y output
% 論理積
function y  = AND(u)
   y = 0;
   dy = true;
   for i = 1:size(u,1)
    dy = logical(u(i)) & dy;
   end
    y = double(dy);
end

== matlab function Control_Logic_e/AND8/AND ==
  data: u input; y output
% 論理積
function y  = AND(u)
   y = 0;
   dy = true;
   for i = 1:size(u,1)
    dy = logical(u(i)) & dy;
   end
    y = double(dy);
end

== matlab function Control_Logic_e/AND7/AND ==
  data: u input; y output
% 論理積
function y  = AND(u)
   y = 0;
   dy = true;
   for i = 1:size(u,1)
    dy = logical(u(i)) & dy;
   end
    y = double(dy);
end

== matlab function Control_Logic_e/AND1/AND ==
  data: u input; y output
% 論理積
function y  = AND(u)
   y = 0;
   dy = true;
   for i = 1:size(u,1)
    dy = logical(u(i)) & dy;
   end
    y = double(dy);
end

== matlab function Control_Logic_e/ANSW1/MATLAB Function ==
  data: u input; y output
% 2位置(アナログ)スイッチ
%   u3入力がONならば、 y=x1(A入力を選択)
%   u3入力がOFFならば、 y=x2(B入力を選択)
%       u(2):A入力変数
%       u(3):B入力変数
%       u3=u(1):C入力変数
%       y : 出力変数
function y  = ANSW(u)
    y = 0;
    temp = logical(u(1));
    temp2 = 0;
    if temp ~= false
        temp2 = u(2);
    else
        temp2 = u(3); 
    end
    y = temp2;
end

== matlab function Control_Logic_e/ANSW2/MATLAB Function ==
  data: u input; y output
% 2位置(アナログ)スイッチ
%   u3入力がONならば、 y=x1(A入力を選択)
%   u3入力がOFFならば、 y=x2(B入力を選択)
%       u(2):A入力変数
%       u(3):B入力変数
%       u3=u(1):C入力変数
%       y : 出力変数
function y  = ANSW(u)
    y = 0;
    temp = logical(u(1));
    temp2 = 0;
    if temp ~= false
        temp2 = u(2);
    else
        temp2 = u(3); 
    end
    y = temp2;
end

== matlab function Control_Logic_e/ABS/ABS ==
  data: u input; y output
function y  = ABS(u)
    y = 0;
    if u(1) > 0
        temp = u(1);
    else
        temp = -u(1);
    end
    y = temp;
end

== matlab function Control_Logic_e/ONDLC7/ONDLC ==
  data: u input; y output; old input
% オンディレイ タイマ
%  xがONとなってからパラメータで設定した[sec]後にyがONとなる。
%  なお、xのON状態がパラメータで設定した[sec]続かずにOFF状態
%  へ戻った場合はyはOFF状態を継続する。
%       ud=u(1) :入力信号
%       set=u(2)：時定数
%       timc(1)=u(3)：計算刻み
%       timc(2)=u(4)：経過時間(前回値)
%       y : 出力信号
function y  = ONDLC(u, old)
       y=zeros(2,1);
       ud = logical(u(1));
       set=u(2);
       timc1=u(3);
       timc2=old(1);
    if ud == false
        temp = false;
        w = 0;
    else
        if timc2 < set 
            temp = false;
            w = timc2 + timc1;
        else
            temp = true;
            w = timc2;
        end
    end
    
    y(1)=double(temp);
    y(2)=w;
end

== matlab function Control_Logic_e/FF1/FF ==
  data: u input; y output; old input
function y  = FF(u,old)
    y = 0;
    set1 = logical(u(1));
    set2 = logical(u(2));
    temp = logical(old(1));
    if (set1 == false) && (set2 == true)
        temp = false;
    else
        if (set1 == true) && (set2 == false)
            temp = true;
        end
    end
    y = double(temp);
end

== matlab function Control_Logic_e/ANSW3/MATLAB Function ==
  data: u input; y output
% 2位置(アナログ)スイッチ
%   u3入力がONならば、 y=x1(A入力を選択)
%   u3入力がOFFならば、 y=x2(B入力を選択)
%       u(2):A入力変数
%       u(3):B入力変数
%       u3=u(1):C入力変数
%       y : 出力変数
function y  = ANSW(u)
    y = 0;
    temp = logical(u(1));
    temp2 = 0;
    if temp ~= false
        temp2 = u(2);
    else
        temp2 = u(3); 
    end
    y = temp2;
end

== matlab function Control_Logic_e/ANSW4/MATLAB Function ==
  data: u input; y output
% 2位置(アナログ)スイッチ
%   u3入力がONならば、 y=x1(A入力を選択)
%   u3入力がOFFならば、 y=x2(B入力を選択)
%       u(2):A入力変数
%       u(3):B入力変数
%       u3=u(1):C入力変数
%       y : 出力変数
function y  = ANSW(u)
    y = 0;
    temp = logical(u(1));
    temp2 = 0;
    if temp ~= false
        temp2 = u(2);
    else
        temp2 = u(3); 
    end
    y = temp2;
end

== matlab function Control_Logic_e/ANSW5/MATLAB Function ==
  data: u input; y output
% 2位置(アナログ)スイッチ
%   u3入力がONならば、 y=x1(A入力を選択)
%   u3入力がOFFならば、 y=x2(B入力を選択)
%       u(2):A入力変数
%       u(3):B入力変数
%       u3=u(1):C入力変数
%       y : 出力変数
function y  = ANSW(u)
    y = 0;
    temp = logical(u(1));
    temp2 = 0;
    if temp ~= false
        temp2 = u(2);
    else
        temp2 = u(3); 
    end
    y = temp2;
end

== matlab function Control_Logic_e/HLM/HLM ==
  data: u input; y output
% 高低モニタ
%   x＞高側設定値ならば、 yをON
%   x＜低側設定値ならば、 yをON
%   上記以外ならばyをOFF
%       u=u(1) :入力変数
%       set(1)=u(1)：低側設定値
%       set(2)=u(3)：高側設定値
%       y : 出力変数
function y  = HLM(u)
    y = 0;
    u1 = u(1);
    set1 = u(2);
    set2 = u(3);
    if (u1 > set1) || (u1 < set2)
        temp= true;
    else
        temp = false; 
    end
    y = double(temp);
end

== matlab function Control_Logic_e/FF/FF ==
  data: u input; y output; old input
function y  = FF(u,old)
    y = 0;
    set1 = logical(u(1));
    set2 = logical(u(2));
    temp = logical(old(1));
    if (set1 == false) && (set2 == true)
        temp = false;
    else
        if (set1 == true) && (set2 == false)
            temp = true;
        end
    end
    y = double(temp);
end

== matlab function Control_Logic_e/OFDLC2/OFDLC ==
  data: u input; y output; old input
% オフディレイ タイマ
%  xがOFFとなってからパラメータで設定した[sec]後にyがOFFとなる。
%  なお、xのOFF状態がパラメータで設定した[sec]続かずにON状態
%  へ戻った場合はyはON状態を継続する。
%       ud=u(1):入力信号
%       set=u(2)：時定数
%       timc(1)=u(3)：計算刻み
%       timc(2)(u4)：経過時間(前回値)
%       y : 出力信号
function y  = OFDLC(u,old)
       y = zeros(2,1);
       ud=logical(u(1));      %:入力信号
       set=u(2);              %：セット時間
       timc1=u(3);          %：計算刻み
       timc2=old(1);          %：経過時間(前回値)

    if ud == true
        temp = true; 
        w = set;
    else
        if timc2 > 0 
            temp = true;
            w = timc2 - timc1;
        else
            temp = false;
            w = timc2;
        end       
    end
    y(1) = double(temp);
    y(2) = w;
end

== matlab function Control_Logic_e/FF2/FF ==
  data: u input; y output; old input
function y  = FF(u,old)
    y = 0;
    set1 = logical(u(1));
    set2 = logical(u(2));
    temp = logical(old(1));
    if (set1 == false) && (set2 == true)
        temp = false;
    else
        if (set1 == true) && (set2 == false)
            temp = true;
        end
    end
    y = double(temp);
end

== matlab function Control_Logic_e/FF4/FF ==
  data: u input; y output; old input
function y  = FF(u,old)
    y = 0;
    set1 = logical(u(1));
    set2 = logical(u(2));
    temp = logical(old(1));
    if (set1 == false) && (set2 == true)
        temp = false;
    else
        if (set1 == true) && (set2 == false)
            temp = true;
        end
    end
    y = double(temp);
end

== matlab function Control_Logic_e/NOT3/NOT ==
  data: u input; y output
%反転
function y  = NOT(u)
    y = 0;
    ud = logical(u(1));
    if ud == false        
        temp = true;
    else
        temp = false;
    end
    y = double(temp);
end

== matlab function Control_Logic_e/FF3/FF ==
  data: u input; y output; old input
function y  = FF(u,old)
    y = 0;
    set1 = logical(u(1));
    set2 = logical(u(2));
    temp = logical(old(1));
    if (set1 == false) && (set2 == true)
        temp = false;
    else
        if (set1 == true) && (set2 == false)
            temp = true;
        end
    end
    y = double(temp);
end

== matlab function Control_Logic_e/AND5/AND ==
  data: u input; y output
% 論理積
function y  = AND(u)
   y = 0;
   dy = true;
   for i = 1:size(u,1)
    dy = logical(u(i)) & dy;
   end
    y = double(dy);
end

== matlab function Control_Logic_e/OFDLC1/OFDLC ==
  data: u input; y output; old input
% オフディレイ タイマ
%  xがOFFとなってからパラメータで設定した[sec]後にyがOFFとなる。
%  なお、xのOFF状態がパラメータで設定した[sec]続かずにON状態
%  へ戻った場合はyはON状態を継続する。
%       ud=u(1):入力信号
%       set=u(2)：時定数
%       timc(1)=u(3)：計算刻み
%       timc(2)(u4)：経過時間(前回値)
%       y : 出力信号
function y  = OFDLC(u,old)
       y = zeros(2,1);
       ud=logical(u(1));      %:入力信号
       set=u(2);              %：セット時間
       timc1=u(3);          %：計算刻み
       timc2=old(1);          %：経過時間(前回値)

    if ud == true
        temp = true; 
        w = set;
    else
        if timc2 > 0 
            temp = true;
            w = timc2 - timc1;
        else
            temp = false;
            w = timc2;
        end       
    end
    y(1) = double(temp);
    y(2) = w;
end

== matlab function Control_Logic_e/OSHOTC/OSHOTC ==
  data: u input; y output; old input; w_old input
% ワンショット タイマ
%  xがOFFからONに変化してからパラメータで設定した[sec]の間、yをONとする。
%  なお、xのON状態がパラメータで設定した[sec]以上継続した場合、あるいは設定以下
%  しか継続しない場合でも、yのON状態の期間はパラメータで設定した時間となる。
%       ud(1) = u(1) ;:入力信号
%       yold = u(2) ;:前回値
%       set = u(3) ;:時定数
%       timc(1) = u(4) ;:計算刻み
%       timc(2) = u(5) ;:経過時間
%       y : 出力信号
function y  = OSHOTC(u,old,w_old)
       y = zeros(2,1);
       ud1 = logical(u(1));
       yold = logical(old(1));
       set = u(2);
       timc1 = u(3);
       timc2 = w_old(1);
       
    if (ud1 == false) && (yold == false)
        w = 0;
        temp = false;
    else
        if set > timc2
            temp = true;
            w = timc2 + timc1;
        else
            temp = false;
            w = timc2;
            if ud1 == false
                w = 0;
            end
        end
    end
    y(1) = double(temp);
    y(2) = w;
end

== matlab function Control_Logic_e/OSHOTC10/OSHOTC ==
  data: u input; y output; old input; w_old input
% ワンショット タイマ
%  xがOFFからONに変化してからパラメータで設定した[sec]の間、yをONとする。
%  なお、xのON状態がパラメータで設定した[sec]以上継続した場合、あるいは設定以下
%  しか継続しない場合でも、yのON状態の期間はパラメータで設定した時間となる。
%       ud(1) = u(1) ;:入力信号
%       yold = u(2) ;:前回値
%       set = u(3) ;:時定数
%       timc(1) = u(4) ;:計算刻み
%       timc(2) = u(5) ;:経過時間
%       y : 出力信号
function y  = OSHOTC(u,old,w_old)
       y = zeros(2,1);
       ud1 = logical(u(1));
       yold = logical(old(1));
       set = u(2);
       timc1 = u(3);
       timc2 = w_old(1);
       
    if (ud1 == false) && (yold == false)
        w = 0;
        temp = false;
    else
        if set > timc2
            temp = true;
            w = timc2 + timc1;
        else
            temp = false;
            w = timc2;
            if ud1 == false
                w = 0;
            end
        end
    end
    y(1) = double(temp);
    y(2) = w;
end

== matlab function Control_Logic_e/OSHOTC12/OSHOTC ==
  data: u input; y output; old input; w_old input
% ワンショット タイマ
%  xがOFFからONに変化してからパラメータで設定した[sec]の間、yをONとする。
%  なお、xのON状態がパラメータで設定した[sec]以上継続した場合、あるいは設定以下
%  しか継続しない場合でも、yのON状態の期間はパラメータで設定した時間となる。
%       ud(1) = u(1) ;:入力信号
%       yold = u(2) ;:前回値
%       set = u(3) ;:時定数
%       timc(1) = u(4) ;:計算刻み
%       timc(2) = u(5) ;:経過時間
%       y : 出力信号
function y  = OSHOTC(u,old,w_old)
       y = zeros(2,1);
       ud1 = logical(u(1));
       yold = logical(old(1));
       set = u(2);
       timc1 = u(3);
       timc2 = w_old(1);
       
    if (ud1 == false) && (yold == false)
        w = 0;
        temp = false;
    else
        if set > timc2
            temp = true;
            w = timc2 + timc1;
        else
            temp = false;
            w = timc2;
            if ud1 == false
                w = 0;
            end
        end
    end
    y(1) = double(temp);
    y(2) = w;
end

== matlab function Control_Logic_e/OSHOTC1/OSHOTC ==
  data: u input; y output; old input; w_old input
% ワンショット タイマ
%  xがOFFからONに変化してからパラメータで設定した[sec]の間、yをONとする。
%  なお、xのON状態がパラメータで設定した[sec]以上継続した場合、あるいは設定以下
%  しか継続しない場合でも、yのON状態の期間はパラメータで設定した時間となる。
%       ud(1) = u(1) ;:入力信号
%       yold = u(2) ;:前回値
%       set = u(3) ;:時定数
%       timc(1) = u(4) ;:計算刻み
%       timc(2) = u(5) ;:経過時間
%       y : 出力信号
function y  = OSHOTC(u,old,w_old)
       y = zeros(2,1);
       ud1 = logical(u(1));
       yold = logical(old(1));
       set = u(2);
       timc1 = u(3);
       timc2 = w_old(1);
       
    if (ud1 == false) && (yold == false)
        w = 0;
        temp = false;
    else
        if set > timc2
            temp = true;
            w = timc2 + timc1;
        else
            temp = false;
            w = timc2;
            if ud1 == false
                w = 0;
            end
        end
    end
    y(1) = double(temp);
    y(2) = w;
end

== matlab function Control_Logic_e/OSHOTC2/OSHOTC ==
  data: u input; y output; old input; w_old input
% ワンショット タイマ
%  xがOFFからONに変化してからパラメータで設定した[sec]の間、yをONとする。
%  なお、xのON状態がパラメータで設定した[sec]以上継続した場合、あるいは設定以下
%  しか継続しない場合でも、yのON状態の期間はパラメータで設定した時間となる。
%       ud(1) = u(1) ;:入力信号
%       yold = u(2) ;:前回値
%       set = u(3) ;:時定数
%       timc(1) = u(4) ;:計算刻み
%       timc(2) = u(5) ;:経過時間
%       y : 出力信号
function y  = OSHOTC(u,old,w_old)
       y = zeros(2,1);
       ud1 = logical(u(1));
       yold = logical(old(1));
       set = u(2);
       timc1 = u(3);
       timc2 = w_old(1);
       
    if (ud1 == false) && (yold == false)
        w = 0;
        temp = false;
    else
        if set > timc2
            temp = true;
            w = timc2 + timc1;
        else
            temp = false;
            w = timc2;
            if ud1 == false
                w = 0;
            end
        end
    end
    y(1) = double(temp);
    y(2) = w;
end

== matlab function Control_Logic_e/NOT/NOT ==
  data: u input; y output
%反転
function y  = NOT(u)
    y = 0;
    ud = logical(u(1));
    if ud == false        
        temp = true;
    else
        temp = false;
    end
    y = double(temp);
end

== matlab function Control_Logic_e/OSHOTC4/OSHOTC ==
  data: u input; y output; old input; w_old input
% ワンショット タイマ
%  xがOFFからONに変化してからパラメータで設定した[sec]の間、yをONとする。
%  なお、xのON状態がパラメータで設定した[sec]以上継続した場合、あるいは設定以下
%  しか継続しない場合でも、yのON状態の期間はパラメータで設定した時間となる。
%       ud(1) = u(1) ;:入力信号
%       yold = u(2) ;:前回値
%       set = u(3) ;:時定数
%       timc(1) = u(4) ;:計算刻み
%       timc(2) = u(5) ;:経過時間
%       y : 出力信号
function y  = OSHOTC(u,old,w_old)
       y = zeros(2,1);
       ud1 = logical(u(1));
       yold = logical(old(1));
       set = u(2);
       timc1 = u(3);
       timc2 = w_old(1);
       
    if (ud1 == false) && (yold == false)
        w = 0;
        temp = false;
    else
        if set > timc2
            temp = true;
            w = timc2 + timc1;
        else
            temp = false;
            w = timc2;
            if ud1 == false
                w = 0;
            end
        end
    end
    y(1) = double(temp);
    y(2) = w;
end

== matlab function Control_Logic_e/OSHOTC3/OSHOTC ==
  data: u input; y output; old input; w_old input
% ワンショット タイマ
%  xがOFFからONに変化してからパラメータで設定した[sec]の間、yをONとする。
%  なお、xのON状態がパラメータで設定した[sec]以上継続した場合、あるいは設定以下
%  しか継続しない場合でも、yのON状態の期間はパラメータで設定した時間となる。
%       ud(1) = u(1) ;:入力信号
%       yold = u(2) ;:前回値
%       set = u(3) ;:時定数
%       timc(1) = u(4) ;:計算刻み
%       timc(2) = u(5) ;:経過時間
%       y : 出力信号
function y  = OSHOTC(u,old,w_old)
       y = zeros(2,1);
       ud1 = logical(u(1));
       yold = logical(old(1));
       set = u(2);
       timc1 = u(3);
       timc2 = w_old(1);
       
    if (ud1 == false) && (yold == false)
        w = 0;
        temp = false;
    else
        if set > timc2
            temp = true;
            w = timc2 + timc1;
        else
            temp = false;
            w = timc2;
            if ud1 == false
                w = 0;
            end
        end
    end
    y(1) = double(temp);
    y(2) = w;
end

== matlab function Control_Logic_e/OSHOTC5/OSHOTC ==
  data: u input; y output; old input; w_old input
% ワンショット タイマ
%  xがOFFからONに変化してからパラメータで設定した[sec]の間、yをONとする。
%  なお、xのON状態がパラメータで設定した[sec]以上継続した場合、あるいは設定以下
%  しか継続しない場合でも、yのON状態の期間はパラメータで設定した時間となる。
%       ud(1) = u(1) ;:入力信号
%       yold = u(2) ;:前回値
%       set = u(3) ;:時定数
%       timc(1) = u(4) ;:計算刻み
%       timc(2) = u(5) ;:経過時間
%       y : 出力信号
function y  = OSHOTC(u,old,w_old)
       y = zeros(2,1);
       ud1 = logical(u(1));
       yold = logical(old(1));
       set = u(2);
       timc1 = u(3);
       timc2 = w_old(1);
       
    if (ud1 == false) && (yold == false)
        w = 0;
        temp = false;
    else
        if set > timc2
            temp = true;
            w = timc2 + timc1;
        else
            temp = false;
            w = timc2;
            if ud1 == false
                w = 0;
            end
        end
    end
    y(1) = double(temp);
    y(2) = w;
end

== matlab function Control_Logic_e/OSHOTC9/OSHOTC ==
  data: u input; y output; old input; w_old input
% ワンショット タイマ
%  xがOFFからONに変化してからパラメータで設定した[sec]の間、yをONとする。
%  なお、xのON状態がパラメータで設定した[sec]以上継続した場合、あるいは設定以下
%  しか継続しない場合でも、yのON状態の期間はパラメータで設定した時間となる。
%       ud(1) = u(1) ;:入力信号
%       yold = u(2) ;:前回値
%       set = u(3) ;:時定数
%       timc(1) = u(4) ;:計算刻み
%       timc(2) = u(5) ;:経過時間
%       y : 出力信号
function y  = OSHOTC(u,old,w_old)
       y = zeros(2,1);
       ud1 = logical(u(1));
       yold = logical(old(1));
       set = u(2);
       timc1 = u(3);
       timc2 = w_old(1);
       
    if (ud1 == false) && (yold == false)
        w = 0;
        temp = false;
    else
        if set > timc2
            temp = true;
            w = timc2 + timc1;
        else
            temp = false;
            w = timc2;
            if ud1 == false
                w = 0;
            end
        end
    end
    y(1) = double(temp);
    y(2) = w;
end

== matlab function Control_Logic_e/ONDLC2/ONDLC ==
  data: u input; y output; old input
% オンディレイ タイマ
%  xがONとなってからパラメータで設定した[sec]後にyがONとなる。
%  なお、xのON状態がパラメータで設定した[sec]続かずにOFF状態
%  へ戻った場合はyはOFF状態を継続する。
%       ud=u(1) :入力信号
%       set=u(2)：時定数
%       timc(1)=u(3)：計算刻み
%       timc(2)=u(4)：経過時間(前回値)
%       y : 出力信号
function y  = ONDLC(u, old)
       y=zeros(2,1);
       ud = logical(u(1));
       set=u(2);
       timc1=u(3);
       timc2=old(1);
    if ud == false
        temp = false;
        w = 0;
    else
        if timc2 < set 
            temp = false;
            w = timc2 + timc1;
        else
            temp = true;
            w = timc2;
        end
    end
    
    y(1)=double(temp);
    y(2)=w;
end
